simulink model "ex_algebraic_loop"  (R2017a)
settings: Solver=ode45  StartTime=0.0  StopTime=10.0  MaxStep=.1  RelTol=1e-3  EnableMultiTasking=on
PreLoadFcn:
  | tau = 1;
settings Model: Creator=The MathWorks, Inc.  LastModifiedBy=sidharth
settings DataIOCC: LimitDataPoints=on  SaveFormat=Array
settings OptimizationCC: ExpressionDepthLimit=2147483647  LifeSpan=inf
settings DebuggingCC: UnderspecifiedInitializationDetection=Classic  MergeDetectMultiDrivingBlocksExec=none  SolverPrmCheckMsg=warning  FcnCallInpInsideContextMsg=warning  StateNameClashWarn=warning  SFUnexpectedBacktrackingDiag=warning  SFNoUnconditionalDefaultTransitionDiag=warning  SFExecutionAtInitializationDiag=none
settings HardwareCC: ProdBitPerPointer=32  ProdBitPerSizeT=32  ProdBitPerPtrDiffT=32  ProdLargestAtomicFloat=None  ProdIntDivRoundTo=Undefined  ProdEndianess=Unspecified  ProdWordSize=32  ProdHWDeviceType=32-bit Generic
settings ModelReferenceCC: PropagateSignalLabelsOutOfModel=off
settings GRTTargetCC: TargetLangStandard=C89/C90 (ANSI)  GeneratePreprocessorConditionals=Disable all  CombineOutputUpdateFcns=off  GRTInterface=on
settings ConfigComp: CovMetricSettings=dw  CovHtmlReporting=on  CovSaveCumulativeToWorkspaceVar=on  CovSaveSingleToWorkspaceVar=on  CovExternalEMLEnable=off

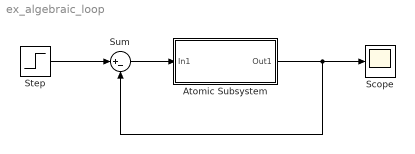
== system ex_algebraic_loop ==
  Atomic Subsystem : Subsystem  TreatAsAtomicUnit=on
  Scope : Scope
  Step : Step  SampleTime=0
  Sum : Sum  Inputs=|+-
  wires:
  Atomic Subsystem/1(Out1) -> Sum/2, Scope/1
  Step/1 -> Sum/1
  Sum/1 -> Atomic Subsystem/1(In1)

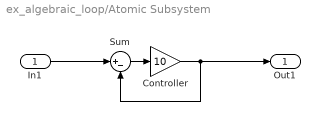
== system ex_algebraic_loop/Atomic Subsystem ==
  In1 : Inport
  Controller : Gain  Gain=10
  Sum : Sum  Inputs=|+-
  Out1 : Outport
  wires:
  Controller/1 -> Out1/1, Sum/2
  In1/1 -> Sum/1
  Sum/1 -> Controller/1
